simulink library "libturbines"  (R2025b)
settings: Solver=ode45  StartTime=0.0  StopTime=10.0  RelTol=1e-3  EnableMultiTasking=on
undefined symbols (not defined in the file): DiscIntNeverNeededParam, dt, faultOptions, noiseFlag
libraries: simulink x57, $bdroot x3
(part 3 of 5)

== system libturbines/Floating NREL5MW faulty/Controller ==
  P_dem [W] : Inport
  w_gen_meas [m/s] : Inport  Port=2
  beta_meas [deg] : Inport  Port=3
  Gain : Gain  Gain=[1 0 0]  Multiplication=Matrix(K*u) (u vector)
  Generator efficiency compensation : Gain  Gain=1/wt.ctrl.gen.effeciency
  Limit power to rated : Saturate  UpperLimit=wt.ctrl.p_rated  LowerLimit=0
  Measurement filter (low pass) : DiscreteStateSpace  A=wt.ctrl.alpha  B=1-wt.ctrl.alpha  C=wt.ctrl.alpha  D=1-wt.ctrl.alpha  InitialCondition=wt.ctrl.gen.ini  SampleTime=wt.ctrl.Ts
  Pitch controller : Subsystem  TreatAsAtomicUnit=on
  Rate Limiter : RateLimiter  RisingSlewLimit=wt.ctrl.torq.ratelim  FallingSlewLimit=-wt.ctrl.torq.ratelim  SampleTimeMode=inherited  InitialCondition=wt.ctrl.torq.ini
  Rated speed : Constant  Value=wt.ctrl.gen.rated
  Region check : Subsystem
  Sample output : ZeroOrderHold  SampleTime=wt.ctrl.Ts
  Sample power demand : ZeroOrderHold  SampleTime=wt.ctrl.Ts
  Saturation : Saturate  UpperLimit=wt.ctrl.torq.lim  LowerLimit=0
  Sum : Sum  Inputs=+-|
  Torque - speed lookup table : Lookup  InputValues=wt.ctrl.torq.wg  Table=wt.ctrl.torq.M  LookUpMeth=Interpolation-Use End Values  SaturateOnIntegerOverflow=off
  Zero-Order Hold : ZeroOrderHold  SampleTime=wt.ctrl.Ts
  beta_ref [deg] : Outport
  T_g_ref [W] : Outport  Port=2
  wires:
  Region check/2(Enable pitch controller) -> Pitch controller/Enable
  Sum/1 -> Pitch controller/1(w_gen_diff)
  Rated speed/1 -> Sum/1
  Sample power demand/1 -> Generator efficiency compensation/1
  Rate Limiter/1 -> Sample output/1
  Generator efficiency compensation/1 -> Limit power to rated/1
  Sample output/1 -> T_g_ref [W]/1
  Zero-Order Hold/1 -> beta_ref [deg]/1
  Limit power to rated/1 -> Region check/3(p_dem), Pitch controller/2(P_dem)
  Region check/1(Torque_ref) -> Saturation/1
  P_dem [W]/1 -> Sample power demand/1
  Torque - speed lookup table/1 -> Region check/1(Torque_dem)  "Desired Torque"
  Pitch controller/1(beta_ref [deg]) -> Gain/1, Zero-Order Hold/1
  Saturation/1 -> Rate Limiter/1
  Measurement filter (low pass)/1 -> Sum/2, Region check/2(w_gen), Torque - speed lookup table/1  "Filtered generator speed"
  w_gen_meas [m/s]/1 -> Measurement filter (low pass)/1
  Gain/1 -> Region check/4(pitch command)
  beta_meas [deg]/1 -> Pitch controller/3(beta_meas [deg])

== system libturbines/Floating NREL5MW faulty/Drive Train ==
  M_rot [Nm] : Inport
  M_gen [Nm] : Inport  Port=2
  Demux : Demux  Outputs=3
  Drive train dynamics : StateSpace  A=wt.dt.ssA  B=wt.dt.ssB  C=wt.dt.ssC  D=wt.dt.ssD  InitialCondition=[wt.rotor.ini;wt.gen.ini;0]
  Mux : Mux  Inputs=2
  w_rot [rad/s] : Outport
  w_gen [rad/s] : Outport  Port=2
  M_shaft [Nm] : Outport  Port=3
  wires:
  Mux/1 -> Drive train dynamics/1
  M_rot [Nm]/1 -> Mux/1
  M_gen [Nm]/1 -> Mux/2
  Drive train dynamics/1 -> Demux/1
  Demux/1 -> w_rot [rad/s]/1
  Demux/2 -> w_gen [rad/s]/1
  Demux/3 -> M_shaft [Nm]/1

== system libturbines/Floating NREL5MW faulty/Generator simple ==
  w_gen [rad/s] : Inport
  T_g_ref [W] : Inport  Port=2
  GenActFault : Inport  Port=3
  Constant : Constant  Value=wt.gen.timeconstant
  Delay : Delay  DelayLength=1  InitialCondition=0
  Delay1 : Delay  DelayLength=1  InitialCondition=0
  Demux : Demux  Outputs=2
  Divide1 : Product  Inputs=*/
  Generator efficiency : Gain  Gain=wt.gen.effeciency
  Generator fault : MATLAB Function  TreatAsAtomicUnit=on
  Generator fault type 3 : MATLAB Function  TreatAsAtomicUnit=on
  Multiply : Product  Inputs=**
  Product : Product
  Sum : Sum  Inputs=|+-
  Torque Integrator : Integrator  InitialCondition=wt.gen.torq.ini
  M_gen [Nm] : Outport
  P_out [W] : Outport  Port=2
  wires:
  Divide1/1 -> Torque Integrator/1
  Generator efficiency/1 -> P_out [W]/1
  Multiply/1 -> Generator efficiency/1
  T_g_ref [W]/1 -> Sum/1
  Torque Integrator/1 -> Generator fault/2(torque), Sum/2
  w_gen [rad/s]/1 -> Multiply/2
  GenActFault/1 -> Generator fault type 3/1(GenActFault)
  Generator fault type 3/1(out) -> Demux/1
  Demux/1 -> Generator fault/1(GenActFault)
  Generator fault/1(torque_real) -> Multiply/1, Delay/1, M_gen [Nm]/1
  Constant/1 -> Product/2
  Demux/2 -> Product/1
  Product/1 -> Divide1/2
  Sum/1 -> Divide1/1
  Delay/1 -> Generator fault/3(torque_prev)
  Generator fault/2(drift_aux_out) -> Delay1/1
  Delay1/1 -> Generator fault/4(drift_aux_in)

== system libturbines/Floating NREL5MW faulty/Hydrodynamics ==
  F_t [N] : Inport
  F_ex : Inport  Port=2
  Gain : Gain  Gain=plat.nF2pT  Multiplication=Matrix(K*u)
  Gain2 : Gain  Gain=plat.pM2nM_surge  Multiplication=Matrix(K*u)
  Gain3 : Gain  Gain=plat.pM2nM_pitch  Multiplication=Matrix(K*u)
  Platform hydrodynamics SS system : StateSpace  A=plat.HydSys.a  B=plat.HydSys.b  C=plat.HydSys.c  D=plat.HydSys.d  InitialCondition=0
  Sum : Sum  Inputs=++|
  Sum2 : Sum  Inputs=+|+
  v_nac_hyd [m/s] : Outport
  wires:
  F_ex/1 -> Sum/2
  Sum/1 -> Platform hydrodynamics SS system/1
  Sum2/1 -> v_nac_hyd [m/s]/1
  Platform hydrodynamics SS system/1 -> Gain3/1, Gain2/1
  Gain2/1 -> Sum2/1
  Gain3/1 -> Sum2/2
  Gain/1 -> Sum/1
  F_t [N]/1 -> Gain/1

== system libturbines/Floating NREL5MW faulty/Pitch Actuator ==
  beta_ref [deg] : Inport
  PitchActFault : Inport  Port=2
  Delay1 : Delay  DelayLength=1  InitialCondition=0
  Delay2 : Delay  DelayLength=1  InitialCondition=0
  Pitch actuator fault : MATLAB Function  TreatAsAtomicUnit=on
  Pitch subsystems : Subsystem
  beta [deg] : Outport
  wires:
  PitchActFault/1 -> Pitch subsystems/2(Fault type 5), Pitch actuator fault/3(PitchActFault)
  beta_ref [deg]/1 -> Pitch subsystems/1(beta_ref [deg])
  Pitch actuator fault/1(beta_real) -> Delay1/1, beta [deg]/1
  Pitch subsystems/1(beta [deg]) -> Pitch actuator fault/1(beta)
  Pitch actuator fault/2(drift_aux_out) -> Delay2/1
  Delay2/1 -> Pitch actuator fault/4(drift_aux_in)
  Delay1/1 -> Pitch actuator fault/2(beta_prev)

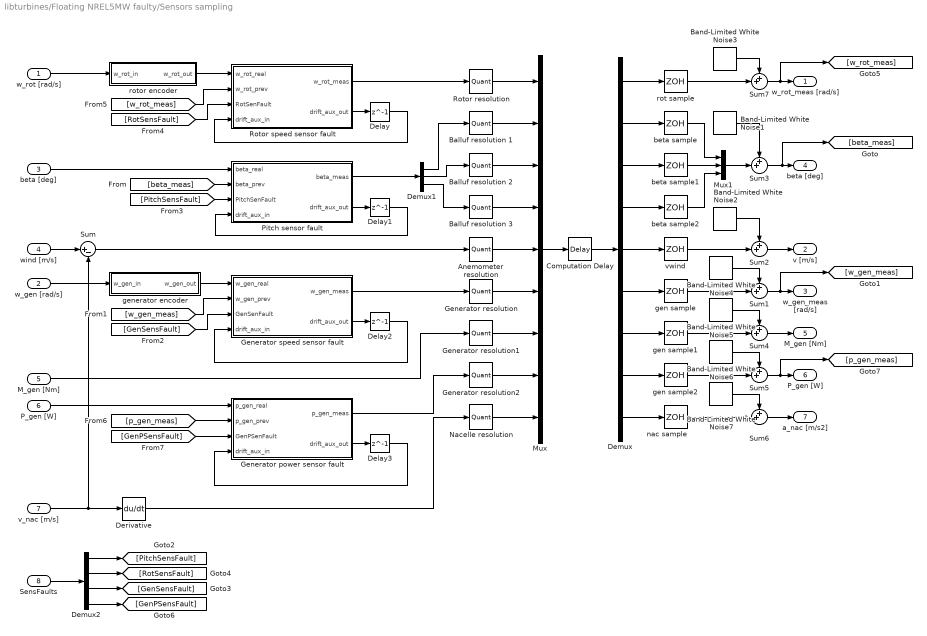
== system libturbines/Floating NREL5MW faulty/Sensors sampling ==
  "w_rot [rad/s] " : Inport
  w_gen [rad/s] : Inport  Port=2
  "beta [deg] " : Inport  Port=3
  wind [m/s] : Inport  Port=4
  "M_gen [Nm] " : Inport  Port=5
  "P_gen [W] " : Inport  Port=6
  "v_nac [m/s] " : Inport  Port=7
  SensFaults : Inport  Port=8
  Anemometer resolution : Quantizer  QuantizationInterval=wt.meas.aneres
  Balluf resolution 1 : Quantizer  QuantizationInterval=wt.meas.pitchres
  Balluf resolution 2 : Quantizer  QuantizationInterval=wt.meas.pitchres
  Balluf resolution 3 : Quantizer  QuantizationInterval=wt.meas.pitchres
  Band-Limited White Noise1 : simulink/Sources/Band-Limited White Noise  Cov=noiseFlag*wt.meas.pitchnoise  Ts=dt  seed=floor(10000*rand(1,3))
  Band-Limited White Noise2 : simulink/Sources/Band-Limited White Noise  Cov=noiseFlag*wt.meas.anenoise  Ts=dt  seed=floor(10000*rand(1))
  Band-Limited White Noise3 : simulink/Sources/Band-Limited White Noise  Cov=noiseFlag*wt.meas.rotSpdnoise  Ts=dt  seed=floor(10000*rand(1))
  Band-Limited White Noise4 : simulink/Sources/Band-Limited White Noise  Cov=noiseFlag*wt.meas.genSpdnoise  Ts=dt  seed=floor(10000*rand(1))
  Band-Limited White Noise5 : simulink/Sources/Band-Limited White Noise  Cov=noiseFlag*wt.meas.genTrqnoise  Ts=dt  seed=floor(10000*rand(1))
  Band-Limited White Noise6 : simulink/Sources/Band-Limited White Noise  Cov=noiseFlag*wt.meas.genPwrnoise  Ts=dt  seed=floor(10000*rand(1))
  Band-Limited White Noise7 : simulink/Sources/Band-Limited White Noise  Cov=noiseFlag*wt.meas.nacAccnoise  Ts=dt  seed=floor(10000*rand(1))
  Computation Delay : TransportDelay  DelayTime=wt.meas.delay  InitialOutput=[wt.rotor.ini wt.pitch.ini wt.pitch.ini wt.pitch.ini 0 wt.gen.ini 0 0 0]
  Delay{,1..3} (4 alike) : Delay  DelayLength=1  InitialCondition=0
  Demux : Demux  Outputs=9
  Demux1 : Demux  Outputs=3
  Demux2 : Demux
  Derivative : Derivative
  Generator power sensor fault : MATLAB Function  TreatAsAtomicUnit=on
  Generator resolution : Quantizer  QuantizationInterval=wt.meas.genres
  Generator resolution1 : Quantizer  QuantizationInterval=wt.meas.genres
  Generator resolution2 : Quantizer  QuantizationInterval=wt.meas.genres
  Generator speed sensor fault : MATLAB Function  TreatAsAtomicUnit=on
  Mux : Mux  Inputs=9
  Mux1 : Mux  Inputs=3
  Nacelle resolution : Quantizer  QuantizationInterval=wt.meas.nacres
  Pitch sensor fault : MATLAB Function  TreatAsAtomicUnit=on
  Rotor resolution : Quantizer  QuantizationInterval=wt.meas.rotres
  Rotor speed sensor fault : MATLAB Function  TreatAsAtomicUnit=on
  Sum : Sum  Inputs=|+-
  Sum{1..7} (7 alike) : Sum  Inputs=++|
  beta sample : ZeroOrderHold  SampleTime=wt.meas.Ts
  beta sample1 : ZeroOrderHold  SampleTime=wt.meas.Ts
  beta sample2 : ZeroOrderHold  SampleTime=wt.meas.Ts
  gen sample : ZeroOrderHold  SampleTime=wt.meas.Ts
  gen sample1 : ZeroOrderHold  SampleTime=wt.meas.Ts
  gen sample2 : ZeroOrderHold  SampleTime=wt.meas.Ts
  generator encoder : Subsystem
  nac sample : ZeroOrderHold  SampleTime=wt.meas.Ts
  rot sample : ZeroOrderHold  SampleTime=wt.meas.Ts
  rotor encoder : Subsystem
  vwind : ZeroOrderHold  SampleTime=wt.meas.Ts
  w_rot_meas [rad/s] : Outport  InitialOutput=0
  v [m/s] : Outport  Port=2  InitialOutput=0
  w_gen_meas [rad/s] : Outport  Port=3  InitialOutput=0
  beta [deg] : Outport  Port=4  InitialOutput=0
  M_gen [Nm] : Outport  Port=5  InitialOutput=0
  P_gen [W] : Outport  Port=6  InitialOutput=0
  a_nac [m/s2] : Outport  Port=7  InitialOutput=0
  wires:
  beta sample1/1 -> Mux1/2
  Demux1/1 -> Balluf resolution 1/1
  Rotor resolution/1 -> Mux/1
  Generator resolution/1 -> Mux/6
  Demux1/2 -> Balluf resolution 2/1
  Demux/6 -> gen sample/1
  Anemometer resolution/1 -> Mux/5
  Demux/5 -> vwind/1
  Mux/1 -> Computation Delay/1
  Computation Delay/1 -> Demux/1
  Demux1/3 -> Balluf resolution 3/1
  beta sample/1 -> Mux1/1
  Demux/1 -> rot sample/1
  beta sample2/1 -> Mux1/3
  Demux/2 -> beta sample/1
  Balluf resolution 1/1 -> Mux/2
  Pitch sensor fault/1(beta_meas) -> Demux1/1
  "beta [deg] "/1 -> Pitch sensor fault/1(beta_real)
  Demux/4 -> beta sample2/1
  Demux/3 -> beta sample1/1
  Balluf resolution 2/1 -> Mux/3
  Balluf resolution 3/1 -> Mux/4
  Generator speed sensor fault/1(w_gen_meas) -> Generator resolution/1
  [w_gen_meas] -> Generator speed sensor fault/2(w_gen_prev)
  [beta_meas] -> Pitch sensor fault/2(beta_prev)
  w_gen [rad/s]/1 -> generator encoder/1(w_gen_in)
  generator encoder/1(w_gen_out) -> Generator speed sensor fault/1(w_gen_real)
  "w_rot [rad/s] "/1 -> rotor encoder/1(w_rot_in)
  Rotor speed sensor fault/1(w_rot_meas) -> Rotor resolution/1
  rotor encoder/1(w_rot_out) -> Rotor speed sensor fault/1(w_rot_real)
  SensFaults/1 -> Demux2/1
  Demux2/1 -> [PitchSensFault]
  [GenSensFault] -> Generator speed sensor fault/3(GenSenFault)
  [PitchSensFault] -> Pitch sensor fault/3(PitchSenFault)
  [RotSensFault] -> Rotor speed sensor fault/3(RotSenFault)
  [w_rot_meas] -> Rotor speed sensor fault/2(w_rot_prev)
  Demux2/2 -> [RotSensFault]
  Demux2/3 -> [GenSensFault]
  Rotor speed sensor fault/2(drift_aux_out) -> Delay/1
  Delay/1 -> Rotor speed sensor fault/4(drift_aux_in)
  Pitch sensor fault/2(drift_aux_out) -> Delay1/1
  Delay1/1 -> Pitch sensor fault/4(drift_aux_in)
  Generator speed sensor fault/2(drift_aux_out) -> Delay2/1
  Delay2/1 -> Generator speed sensor fault/4(drift_aux_in)
  "M_gen [Nm] "/1 -> Generator resolution1/1
  "v_nac [m/s] "/1 -> Derivative/1, Sum/2
  Derivative/1 -> Nacelle resolution/1
  Generator resolution1/1 -> Mux/7
  Nacelle resolution/1 -> Mux/9
  Generator resolution2/1 -> Mux/8
  Band-Limited White Noise5/1 -> Sum4/1
  Sum4/1 -> M_gen [Nm]/1
  Sum6/1 -> a_nac [m/s2]/1
  Band-Limited White Noise7/1 -> Sum6/1
  Band-Limited White Noise6/1 -> Sum5/1
  nac sample/1 -> Sum6/2
  gen sample1/1 -> Sum4/2
  Sum5/1 -> [p_gen_meas], P_gen [W]/1
  gen sample2/1 -> Sum5/2
  Demux/7 -> gen sample1/1
  Demux/8 -> gen sample2/1
  Demux/9 -> nac sample/1
  Sum1/1 -> [w_gen_meas], w_gen_meas [rad/s]/1
  gen sample/1 -> Sum1/2
  Sum2/1 -> v [m/s]/1
  vwind/1 -> Sum2/2
  Mux1/1 -> Sum3/2
  Sum3/1 -> [beta_meas], beta [deg]/1
  rot sample/1 -> Sum7/2
  Sum7/1 -> [w_rot_meas], w_rot_meas [rad/s]/1
  Band-Limited White Noise4/1 -> Sum1/1
  Band-Limited White Noise2/1 -> Sum2/1
  Band-Limited White Noise1/1 -> Sum3/1
  Band-Limited White Noise3/1 -> Sum7/1
  Sum/1 -> Anemometer resolution/1
  wind [m/s]/1 -> Sum/1
  Demux2/4 -> [GenPSensFault]
  Delay3/1 -> Generator power sensor fault/4(drift_aux_in)
  [GenPSensFault] -> Generator power sensor fault/3(GenPSenFault)
  Generator power sensor fault/2(drift_aux_out) -> Delay3/1
  "P_gen [W] "/1 -> Generator power sensor fault/1(p_gen_real)
  Generator power sensor fault/1(p_gen_meas) -> Generator resolution2/1
  [p_gen_meas] -> Generator power sensor fault/2(p_gen_prev)

== system libturbines/Floating NREL5MW faulty/Tower deflection  ==
  F_t [N] : Inport
  F_t*h : Gain  Gain=wt.tower.height  SaturateOnIntegerOverflow=on  OutDataTypeStr=Inherit: Same as input  ParamDataTypeStr=Inherit: Same as input
  Tower1 : Subsystem  mask(Tower (thrustwise)){mtop=wt.top.mass, mtow=wt.tower.mass, ftowY=wt.tower.eigfreq, dampY=wt.tower.damp}
      mask prompts: mtop "Mass of towertop [kg]"; mtow "Aequivalent tower mass [kg]"; ftowY "Tower eigenfrequency [Hz]"; dampY "Damping coefficient"
      mask help: Thrustwise dynamics of the tower
      mask init: same as libturbines/Floating IEA15MW/Tower /Tower1
      mask Help: The thrustwise tower dynamics are modelled as a linear oscillator
  v_nac [m/s] : Outport
  M_tow [Nm] : Outport  Port=2
  wires:
  Tower1/2(F_tow [N]) -> F_t*h/1
  F_t*h/1 -> M_tow [Nm]/1
  F_t [N]/1 -> Tower1/1(FT [Nm])
  Tower1/1(vnac [m/s]) -> v_nac [m/s]/1

== system libturbines/Floating IEA15MW/Controller/Pitch controller ==
  w_gen_diff : Inport
  P_dem : Inport  Port=2
  beta_meas [deg] : Inport  Port=3
  Enable : EnablePort  StatesWhenEnabling=reset  PropagateVarSize=During execution
  Blade 1 controller : Subsystem
  beta_ref [deg] : Outport  OutputWhenDisabled=reset  InitialOutput=wt.ctrl.torq.beta
  wires:
  Blade 1 controller/1(beta_ref [deg]) -> beta_ref [deg]/1
  beta_meas [deg]/1 -> Blade 1 controller/3(beta_meas [deg])
  P_dem/1 -> Blade 1 controller/2(P_dem)
  w_gen_diff/1 -> Blade 1 controller/1(w_gen_diff)

== system libturbines/Floating IEA15MW/Controller/Region check ==
  Torque_dem : Inport
  w_gen : Inport  Port=2
  p_dem : Inport  Port=3
  pitch command : Inport  Port=4
  Demand limitation : RelationalOperator  Operator=<=  OutDataTypeStr=boolean  InputSameDT=off
  Divide : Product  Inputs=*/
  Enable Pitch control? : Logic  Operator=OR  Inputs=3  AllPortsSameDT=off  OutDataTypeStr=boolean
  Integer Delay : Delay  DelayLength=1
  Pitch actuator active last time? : simulink/Logic and Bit Operations/Compare To Constant  relop=>  const=wt.ctrl.torq.beta  OutDataTypeStr=uint8  ZeroCross=off
  Product : Product  RndMeth=Zero
  Region 3 speed? : simulink/Logic and Bit Operations/Compare To Constant  relop=>=  const=wt.ctrl.torq.r3  OutDataTypeStr=uint8  ZeroCross=off
  Switch Torque_ref : Switch  Threshold=1  SaturateOnIntegerOverflow=off  InputSameDT=off
  Torque_ref : Outport
  Enable pitch controller : Outport  Port=2
  wires:
  Divide/1 -> Switch Torque_ref/1
  Switch Torque_ref/1 -> Torque_ref/1
  Demand limitation/1 -> Enable Pitch control?/1
  p_dem/1 -> Divide/1, Demand limitation/1
  Torque_dem/1 -> Switch Torque_ref/3, Product/1
  Product/1 -> Demand limitation/2
  Enable Pitch control?/1 -> Switch Torque_ref/2, Enable pitch controller/1
  Integer Delay/1 -> Pitch actuator active last time?/1
  Region 3 speed?/1 -> Enable Pitch control?/2
  Pitch actuator active last time?/1 -> Enable Pitch control?/3
  w_gen/1 -> Product/2, Region 3 speed?/1, Divide/2
  pitch command/1 -> Integer Delay/1

== system libturbines/Floating IEA15MW/Sensors sampling/generator encoder ==
  w_gen_in : Inport
  Sum : Sum  Inputs=-+|
  gen Integrator : Integrator  InitialCondition=wt.gen.ini
  gen sensor time constant : Gain  Gain=1/wt.meas.gentau
  w_gen_out : Outport
  wires:
  gen Integrator/1 -> w_gen_out/1, Sum/1
  Sum/1 -> gen sensor time constant/1
  gen sensor time constant/1 -> gen Integrator/1
  w_gen_in/1 -> Sum/2

== system libturbines/Floating IEA15MW/Sensors sampling/rotor encoder ==
  w_rot_in : Inport
  Sum1 : Sum  Inputs=|+-
  gen Integrator1 : Integrator  InitialCondition=wt.rotor.ini
  gen sensor time constant1 : Gain  Gain=1/wt.meas.rottau
  w_rot_out : Outport
  wires:
  w_rot_in/1 -> Sum1/1
  gen Integrator1/1 -> w_rot_out/1, Sum1/2
  Sum1/1 -> gen sensor time constant1/1
  gen sensor time constant1/1 -> gen Integrator1/1

== system libturbines/Floating IEA15MW/Tower /Tower1 ==
  FT [Nm] : Inport
  Demux1 : Demux  Outputs=2
  Tower : StateSpace  A=A  B=B  C=C  D=D  InitialCondition=zeros(2,1)
  vnac [m/s] : Outport  InitialOutput=0
  F_tow [N] : Outport  Port=2  InitialOutput=0
  wires:
  Demux1/2 -> F_tow [N]/1
  FT [Nm]/1 -> Tower/1
  Demux1/1 -> vnac [m/s]/1
  Tower/1 -> Demux1/1

== system libturbines/Floating IEA15MW faulty/Aerodynamics/Blade 1 ==
  note: tip speed
      | [m/s]
  v_rot [m/s] : Inport
  beta [deg] : Inport  Port=2
  w_rot [rad/s] : Inport  Port=3
  C_P & C_T tables : Subsystem
  Gain : Gain  Gain=1/3
  Gain1 : Gain  Gain=1/3
  Gain2 : Gain  Gain=1/3
  Math Function : Math  Operator=square  SignedPower=on
  Product : Product  InputSameDT=on  SaturateOnIntegerOverflow=on  OutDataTypeStr=Inherit: Same as first input
  Product1 : Product  Inputs=**/  InputSameDT=on  SaturateOnIntegerOverflow=on  OutDataTypeStr=Inherit: Same as first input
  Product2 : Product  InputSameDT=on  SaturateOnIntegerOverflow=on  OutDataTypeStr=Inherit: Same as first input
  Product3 : Product  Inputs=/*  InputSameDT=on  SaturateOnIntegerOverflow=on  OutDataTypeStr=Inherit: Same as first input
  rho/2*A : Gain  Gain=env.rho*.5* pi * wt.rotor.radius^2  SaturateOnIntegerOverflow=on  OutDataTypeStr=Inherit: Same as input  ParamDataTypeStr=Inherit: Same as input
  rotor radius : Gain  Gain=wt.rotor.radius  SaturateOnIntegerOverflow=on  OutDataTypeStr=Inherit: Same as input  ParamDataTypeStr=Inherit: Same as input
  F_t [N] : Outport
  C_T : Outport  Port=2
  M_rot [Nm] : Outport  Port=3
  wires:
  Gain1/1 -> C_T/1
  Gain2/1 -> M_rot [Nm]/1
  Gain/1 -> F_t [N]/1
  Product/1 -> Gain/1
  Product1/1 -> Gain2/1
  beta [deg]/1 -> C_P & C_T tables/1(beta)
  Math Function/1 -> rho/2*A/1
  rotor radius/1 -> Product3/2
  v_rot [m/s]/1 -> Math Function/1, Product3/1, Product2/1
  w_rot [rad/s]/1 -> rotor radius/1, Product1/3
  Product2/1 -> Product1/2
  rho/2*A/1 -> Product2/2, Product/1
  Product3/1 -> C_P & C_T tables/2(lambda)
  C_P & C_T tables/1(C_T) -> Product/2, Gain1/1
  C_P & C_T tables/2(C_P) -> Product1/1

== system libturbines/Floating IEA15MW faulty/Aerodynamics/Blade 2 ==
  note: tip speed
      | [m/s]
  v_rot [m/s] : Inport
  beta [deg] : Inport  Port=2
  w_rot [rad/s] : Inport  Port=3
  C_P & C_T tables : Subsystem
  Gain : Gain  Gain=1/3
  Gain1 : Gain  Gain=1/3
  Gain2 : Gain  Gain=1/3
  Math Function : Math  Operator=square  SignedPower=on
  Product : Product  InputSameDT=on  SaturateOnIntegerOverflow=on  OutDataTypeStr=Inherit: Same as first input
  Product1 : Product  Inputs=**/  InputSameDT=on  SaturateOnIntegerOverflow=on  OutDataTypeStr=Inherit: Same as first input
  Product2 : Product  InputSameDT=on  SaturateOnIntegerOverflow=on  OutDataTypeStr=Inherit: Same as first input
  Product3 : Product  Inputs=/*  InputSameDT=on  SaturateOnIntegerOverflow=on  OutDataTypeStr=Inherit: Same as first input
  rho/2*A : Gain  Gain=env.rho*.5* pi * wt.rotor.radius^2  SaturateOnIntegerOverflow=on  OutDataTypeStr=Inherit: Same as input  ParamDataTypeStr=Inherit: Same as input
  rotor radius : Gain  Gain=wt.rotor.radius  SaturateOnIntegerOverflow=on  OutDataTypeStr=Inherit: Same as input  ParamDataTypeStr=Inherit: Same as input
  F_t [N] : Outport
  C_T : Outport  Port=2
  M_rot [Nm] : Outport  Port=3
  wires:
  Gain1/1 -> C_T/1
  Gain2/1 -> M_rot [Nm]/1
  Gain/1 -> F_t [N]/1
  Product/1 -> Gain/1
  Product1/1 -> Gain2/1
  beta [deg]/1 -> C_P & C_T tables/1(beta)
  Math Function/1 -> rho/2*A/1
  rotor radius/1 -> Product3/2
  v_rot [m/s]/1 -> Math Function/1, Product3/1, Product2/1
  w_rot [rad/s]/1 -> rotor radius/1, Product1/3
  Product2/1 -> Product1/2
  rho/2*A/1 -> Product2/2, Product/1
  Product3/1 -> C_P & C_T tables/2(lambda)
  C_P & C_T tables/1(C_T) -> Product/2, Gain1/1
  C_P & C_T tables/2(C_P) -> Product1/1

== system libturbines/Floating IEA15MW faulty/Aerodynamics/Blade 3 ==
  note: tip speed
      | [m/s]
  v_rot [m/s] : Inport
  beta [deg] : Inport  Port=2
  w_rot [rad/s] : Inport  Port=3
  C_P & C_T tables : Subsystem
  Gain : Gain  Gain=1/3
  Gain1 : Gain  Gain=1/3
  Gain2 : Gain  Gain=1/3
  Math Function : Math  Operator=square  SignedPower=on
  Product : Product  InputSameDT=on  SaturateOnIntegerOverflow=on  OutDataTypeStr=Inherit: Same as first input
  Product1 : Product  Inputs=**/  InputSameDT=on  SaturateOnIntegerOverflow=on  OutDataTypeStr=Inherit: Same as first input
  Product2 : Product  InputSameDT=on  SaturateOnIntegerOverflow=on  OutDataTypeStr=Inherit: Same as first input
  Product3 : Product  Inputs=/*  InputSameDT=on  SaturateOnIntegerOverflow=on  OutDataTypeStr=Inherit: Same as first input
  rho/2*A : Gain  Gain=env.rho*.5* pi * wt.rotor.radius^2  SaturateOnIntegerOverflow=on  OutDataTypeStr=Inherit: Same as input  ParamDataTypeStr=Inherit: Same as input
  rotor radius : Gain  Gain=wt.rotor.radius  SaturateOnIntegerOverflow=on  OutDataTypeStr=Inherit: Same as input  ParamDataTypeStr=Inherit: Same as input
  F_t [N] : Outport
  C_T : Outport  Port=2
  M_rot [Nm] : Outport  Port=3
  wires:
  Gain1/1 -> C_T/1
  Gain2/1 -> M_rot [Nm]/1
  Gain/1 -> F_t [N]/1
  Product/1 -> Gain/1
  Product1/1 -> Gain2/1
  beta [deg]/1 -> C_P & C_T tables/1(beta)
  Math Function/1 -> rho/2*A/1
  rotor radius/1 -> Product3/2
  v_rot [m/s]/1 -> Math Function/1, Product3/1, Product2/1
  w_rot [rad/s]/1 -> rotor radius/1, Product1/3
  Product2/1 -> Product1/2
  rho/2*A/1 -> Product2/2, Product/1
  Product3/1 -> C_P & C_T tables/2(lambda)
  C_P & C_T tables/1(C_T) -> Product/2, Gain1/1
  C_P & C_T tables/2(C_P) -> Product1/1

== system libturbines/Floating IEA15MW faulty/Controller/Pitch controller ==
  w_gen_diff : Inport
  P_dem : Inport  Port=2
  beta_meas [deg] : Inport  Port=3
  Enable : EnablePort  StatesWhenEnabling=reset  PropagateVarSize=During execution
  Blade 1 controller : Subsystem
  Blade 2 controller : Subsystem
  Blade 3 controller : Subsystem
  Demux : Demux  Outputs=3
  Mux : Mux  Inputs=3
  beta_ref [deg] : Outport  OutputWhenDisabled=reset  InitialOutput=wt.ctrl.torq.beta
  wires:
  Mux/1 -> beta_ref [deg]/1
  w_gen_diff/1 -> Blade 1 controller/1(w_gen_diff), Blade 2 controller/1(w_gen_diff), Blade 3 controller/1(w_gen_diff)
  P_dem/1 -> Blade 1 controller/2(P_dem), Blade 2 controller/2(P_dem), Blade 3 controller/2(P_dem)
  Demux/1 -> Blade 1 controller/3(beta_meas [deg])
  Blade 1 controller/1(beta_ref [deg]) -> Mux/1
  Demux/2 -> Blade 2 controller/3(beta_meas [deg])
  beta_meas [deg]/1 -> Demux/1
  Blade 3 controller/1(beta_ref [deg]) -> Mux/3
  Demux/3 -> Blade 3 controller/3(beta_meas [deg])
  Blade 2 controller/1(beta_ref [deg]) -> Mux/2

== system libturbines/Floating IEA15MW faulty/Controller/Region check ==
  Torque_dem : Inport
  w_gen : Inport  Port=2
  p_dem : Inport  Port=3
  pitch command : Inport  Port=4
  Demand limitation : RelationalOperator  Operator=<=  OutDataTypeStr=boolean  InputSameDT=off
  Divide : Product  Inputs=*/
  Enable Pitch control? : Logic  Operator=OR  Inputs=3  AllPortsSameDT=off  OutDataTypeStr=boolean
  Integer Delay : Delay  DelayLength=1
  Pitch actuator active last time? : simulink/Logic and Bit Operations/Compare To Constant  relop=>  const=wt.ctrl.torq.beta  OutDataTypeStr=uint8  ZeroCross=off
  Product : Product  RndMeth=Zero
  Region 3 speed? : simulink/Logic and Bit Operations/Compare To Constant  relop=>=  const=wt.ctrl.torq.r3  OutDataTypeStr=uint8  ZeroCross=off
  Switch Torque_ref : Switch  Threshold=1  SaturateOnIntegerOverflow=off  InputSameDT=off
  Torque_ref : Outport
  Enable pitch controller : Outport  Port=2
  wires:
  pitch command/1 -> Integer Delay/1
  w_gen/1 -> Divide/2, Region 3 speed?/1, Product/2
  Pitch actuator active last time?/1 -> Enable Pitch control?/3
  Region 3 speed?/1 -> Enable Pitch control?/2
  Integer Delay/1 -> Pitch actuator active last time?/1
  Enable Pitch control?/1 -> Enable pitch controller/1, Switch Torque_ref/2
  Product/1 -> Demand limitation/2
  Torque_dem/1 -> Product/1, Switch Torque_ref/3
  p_dem/1 -> Demand limitation/1, Divide/1
  Demand limitation/1 -> Enable Pitch control?/1
  Switch Torque_ref/1 -> Torque_ref/1
  Divide/1 -> Switch Torque_ref/1

== system libturbines/Floating IEA15MW faulty/Pitch Actuator/Pitch subsystems ==
  beta_ref [deg] : Inport
  Fault type 5 : Inport  Port=2
  Demux2 : Demux  Outputs=3
  Mux1 : Mux  Inputs=3
  Pitch system B1 : StateSpace  A=wt.pitch.ssA  B=wt.pitch.ssB  C=wt.pitch.ssC  D=wt.pitch.ssD  InitialCondition=0
  Pitch system B2 : StateSpace  A=wt.pitch.ssA  B=wt.pitch.ssB  C=wt.pitch.ssC  D=wt.pitch.ssD  InitialCondition=0
  Pitch system B3 : Subsystem
  beta [deg] : Outport
  wires:
  Demux2/2 -> Pitch system B2/1
  Demux2/1 -> Pitch system B1/1
  Pitch system B1/1 -> Mux1/1
  Pitch system B2/1 -> Mux1/2
  Mux1/1 -> beta [deg]/1
  beta_ref [deg]/1 -> Demux2/1
  Fault type 5/1 -> Pitch system B3/2(fault 5)
  Demux2/3 -> Pitch system B3/1(beta_ref [deg])
  Pitch system B3/1(beta [deg]) -> Mux1/3

== system libturbines/Floating IEA15MW faulty/Sensors sampling/generator encoder ==
  w_gen_in : Inport
  Sum : Sum  Inputs=-+|
  gen Integrator : Integrator  InitialCondition=wt.gen.ini
  gen sensor time constant : Gain  Gain=1/wt.meas.gentau
  w_gen_out : Outport
  wires:
  w_gen_in/1 -> Sum/2
  gen sensor time constant/1 -> gen Integrator/1
  Sum/1 -> gen sensor time constant/1
  gen Integrator/1 -> Sum/1, w_gen_out/1

== system libturbines/Floating IEA15MW faulty/Sensors sampling/rotor encoder ==
  w_rot_in : Inport
  Sum1 : Sum  Inputs=|+-
  gen Integrator1 : Integrator  InitialCondition=wt.rotor.ini
  gen sensor time constant1 : Gain  Gain=1/wt.meas.rottau
  w_rot_out : Outport
  wires:
  gen sensor time constant1/1 -> gen Integrator1/1
  Sum1/1 -> gen sensor time constant1/1
  gen Integrator1/1 -> Sum1/2, w_rot_out/1
  w_rot_in/1 -> Sum1/1

== system libturbines/Floating IEA15MW faulty/Tower deflection /Tower1 ==
  FT [Nm] : Inport
  Demux1 : Demux  Outputs=2
  Tower : StateSpace  A=A  B=B  C=C  D=D  InitialCondition=zeros(2,1)
  vnac [m/s] : Outport  InitialOutput=0
  F_tow [N] : Outport  Port=2  InitialOutput=0
  wires:
  Tower/1 -> Demux1/1
  Demux1/1 -> vnac [m/s]/1
  FT [Nm]/1 -> Tower/1
  Demux1/2 -> F_tow [N]/1

== system libturbines/Floating IEA3.4MW/Controller/Pitch controller ==
  w_gen_diff : Inport
  P_dem : Inport  Port=2
  beta_meas [deg] : Inport  Port=3
  Enable : EnablePort  StatesWhenEnabling=reset  PropagateVarSize=During execution
  Blade 1 controller : Subsystem
  beta_ref [deg] : Outport  OutputWhenDisabled=reset  InitialOutput=wt.ctrl.torq.beta
  wires:
  Blade 1 controller/1(beta_ref [deg]) -> beta_ref [deg]/1
  beta_meas [deg]/1 -> Blade 1 controller/3(beta_meas [deg])
  P_dem/1 -> Blade 1 controller/2(P_dem)
  w_gen_diff/1 -> Blade 1 controller/1(w_gen_diff)

== system libturbines/Floating IEA3.4MW/Controller/Region check ==
  Torque_dem : Inport
  w_gen : Inport  Port=2
  p_dem : Inport  Port=3
  pitch command : Inport  Port=4
  Demand limitation : RelationalOperator  Operator=<=  OutDataTypeStr=boolean  InputSameDT=off
  Divide : Product  Inputs=*/
  Enable Pitch control? : Logic  Operator=OR  Inputs=3  AllPortsSameDT=off  OutDataTypeStr=boolean
  Integer Delay : Delay  DelayLength=1
  Pitch actuator active last time? : simulink/Logic and Bit Operations/Compare To Constant  relop=>  const=wt.ctrl.torq.beta  OutDataTypeStr=uint8  ZeroCross=off
  Product : Product  RndMeth=Zero
  Region 3 speed? : simulink/Logic and Bit Operations/Compare To Constant  relop=>=  const=wt.ctrl.torq.r3  OutDataTypeStr=uint8  ZeroCross=off
  Switch Torque_ref : Switch  Threshold=1  SaturateOnIntegerOverflow=off  InputSameDT=off
  Torque_ref : Outport
  Enable pitch controller : Outport  Port=2
  wires:
  Divide/1 -> Switch Torque_ref/1
  Switch Torque_ref/1 -> Torque_ref/1
  Demand limitation/1 -> Enable Pitch control?/1
  p_dem/1 -> Divide/1, Demand limitation/1
  Torque_dem/1 -> Switch Torque_ref/3, Product/1
  Product/1 -> Demand limitation/2
  Enable Pitch control?/1 -> Switch Torque_ref/2, Enable pitch controller/1
  Integer Delay/1 -> Pitch actuator active last time?/1
  Region 3 speed?/1 -> Enable Pitch control?/2
  Pitch actuator active last time?/1 -> Enable Pitch control?/3
  w_gen/1 -> Product/2, Region 3 speed?/1, Divide/2
  pitch command/1 -> Integer Delay/1

== system libturbines/Floating IEA3.4MW/Sensors sampling/generator encoder ==
  w_gen_in : Inport
  Sum : Sum  Inputs=-+|
  gen Integrator : Integrator  InitialCondition=wt.gen.ini
  gen sensor time constant : Gain  Gain=1/wt.meas.gentau
  w_gen_out : Outport
  wires:
  gen Integrator/1 -> w_gen_out/1, Sum/1
  Sum/1 -> gen sensor time constant/1
  gen sensor time constant/1 -> gen Integrator/1
  w_gen_in/1 -> Sum/2

== system libturbines/Floating IEA3.4MW/Sensors sampling/rotor encoder ==
  w_rot_in : Inport
  Sum1 : Sum  Inputs=|+-
  gen Integrator1 : Integrator  InitialCondition=wt.rotor.ini
  gen sensor time constant1 : Gain  Gain=1/wt.meas.rottau
  w_rot_out : Outport
  wires:
  w_rot_in/1 -> Sum1/1
  gen Integrator1/1 -> w_rot_out/1, Sum1/2
  Sum1/1 -> gen sensor time constant1/1
  gen sensor time constant1/1 -> gen Integrator1/1

== system libturbines/Floating IEA3.4MW/Tower /Tower1 ==
  FT [Nm] : Inport
  Demux1 : Demux  Outputs=2
  Tower : StateSpace  A=A  B=B  C=C  D=D  InitialCondition=zeros(2,1)
  vnac [m/s] : Outport  InitialOutput=0
  F_tow [N] : Outport  Port=2  InitialOutput=0
  wires:
  Demux1/2 -> F_tow [N]/1
  FT [Nm]/1 -> Tower/1
  Demux1/1 -> vnac [m/s]/1
  Tower/1 -> Demux1/1

== system libturbines/Floating IEA3.4MW faulty/Aerodynamics/Blade 1 ==
  note: tip speed
      | [m/s]
  v_rot [m/s] : Inport
  beta [deg] : Inport  Port=2
  w_rot [rad/s] : Inport  Port=3
  C_P & C_T tables : Subsystem
  Gain : Gain  Gain=1/3
  Gain1 : Gain  Gain=1/3
  Gain2 : Gain  Gain=1/3
  Math Function : Math  Operator=square  SignedPower=on
  Product : Product  InputSameDT=on  SaturateOnIntegerOverflow=on  OutDataTypeStr=Inherit: Same as first input
  Product1 : Product  Inputs=**/  InputSameDT=on  SaturateOnIntegerOverflow=on  OutDataTypeStr=Inherit: Same as first input
  Product2 : Product  InputSameDT=on  SaturateOnIntegerOverflow=on  OutDataTypeStr=Inherit: Same as first input
  Product3 : Product  Inputs=/*  InputSameDT=on  SaturateOnIntegerOverflow=on  OutDataTypeStr=Inherit: Same as first input
  rho/2*A : Gain  Gain=env.rho*.5* pi * wt.rotor.radius^2  SaturateOnIntegerOverflow=on  OutDataTypeStr=Inherit: Same as input  ParamDataTypeStr=Inherit: Same as input
  rotor radius : Gain  Gain=wt.rotor.radius  SaturateOnIntegerOverflow=on  OutDataTypeStr=Inherit: Same as input  ParamDataTypeStr=Inherit: Same as input
  F_t [N] : Outport
  C_T : Outport  Port=2
  M_rot [Nm] : Outport  Port=3
  wires:
  Gain1/1 -> C_T/1
  Gain2/1 -> M_rot [Nm]/1
  Gain/1 -> F_t [N]/1
  Product/1 -> Gain/1
  Product1/1 -> Gain2/1
  beta [deg]/1 -> C_P & C_T tables/1(beta)
  Math Function/1 -> rho/2*A/1
  rotor radius/1 -> Product3/2
  v_rot [m/s]/1 -> Math Function/1, Product3/1, Product2/1
  w_rot [rad/s]/1 -> rotor radius/1, Product1/3
  Product2/1 -> Product1/2
  rho/2*A/1 -> Product2/2, Product/1
  Product3/1 -> C_P & C_T tables/2(lambda)
  C_P & C_T tables/1(C_T) -> Product/2, Gain1/1
  C_P & C_T tables/2(C_P) -> Product1/1

== system libturbines/Floating IEA3.4MW faulty/Aerodynamics/Blade 2 ==
  note: tip speed
      | [m/s]
  v_rot [m/s] : Inport
  beta [deg] : Inport  Port=2
  w_rot [rad/s] : Inport  Port=3
  C_P & C_T tables : Subsystem
  Gain : Gain  Gain=1/3
  Gain1 : Gain  Gain=1/3
  Gain2 : Gain  Gain=1/3
  Math Function : Math  Operator=square  SignedPower=on
  Product : Product  InputSameDT=on  SaturateOnIntegerOverflow=on  OutDataTypeStr=Inherit: Same as first input
  Product1 : Product  Inputs=**/  InputSameDT=on  SaturateOnIntegerOverflow=on  OutDataTypeStr=Inherit: Same as first input
  Product2 : Product  InputSameDT=on  SaturateOnIntegerOverflow=on  OutDataTypeStr=Inherit: Same as first input
  Product3 : Product  Inputs=/*  InputSameDT=on  SaturateOnIntegerOverflow=on  OutDataTypeStr=Inherit: Same as first input
  rho/2*A : Gain  Gain=env.rho*.5* pi * wt.rotor.radius^2  SaturateOnIntegerOverflow=on  OutDataTypeStr=Inherit: Same as input  ParamDataTypeStr=Inherit: Same as input
  rotor radius : Gain  Gain=wt.rotor.radius  SaturateOnIntegerOverflow=on  OutDataTypeStr=Inherit: Same as input  ParamDataTypeStr=Inherit: Same as input
  F_t [N] : Outport
  C_T : Outport  Port=2
  M_rot [Nm] : Outport  Port=3
  wires:
  Gain1/1 -> C_T/1
  Gain2/1 -> M_rot [Nm]/1
  Gain/1 -> F_t [N]/1
  Product/1 -> Gain/1
  Product1/1 -> Gain2/1
  beta [deg]/1 -> C_P & C_T tables/1(beta)
  Math Function/1 -> rho/2*A/1
  rotor radius/1 -> Product3/2
  v_rot [m/s]/1 -> Math Function/1, Product3/1, Product2/1
  w_rot [rad/s]/1 -> rotor radius/1, Product1/3
  Product2/1 -> Product1/2
  rho/2*A/1 -> Product2/2, Product/1
  Product3/1 -> C_P & C_T tables/2(lambda)
  C_P & C_T tables/1(C_T) -> Product/2, Gain1/1
  C_P & C_T tables/2(C_P) -> Product1/1

== system libturbines/Floating IEA3.4MW faulty/Aerodynamics/Blade 3 ==
  note: tip speed
      | [m/s]
  v_rot [m/s] : Inport
  beta [deg] : Inport  Port=2
  w_rot [rad/s] : Inport  Port=3
  C_P & C_T tables : Subsystem
  Gain : Gain  Gain=1/3
  Gain1 : Gain  Gain=1/3
  Gain2 : Gain  Gain=1/3
  Math Function : Math  Operator=square  SignedPower=on
  Product : Product  InputSameDT=on  SaturateOnIntegerOverflow=on  OutDataTypeStr=Inherit: Same as first input
  Product1 : Product  Inputs=**/  InputSameDT=on  SaturateOnIntegerOverflow=on  OutDataTypeStr=Inherit: Same as first input
  Product2 : Product  InputSameDT=on  SaturateOnIntegerOverflow=on  OutDataTypeStr=Inherit: Same as first input
  Product3 : Product  Inputs=/*  InputSameDT=on  SaturateOnIntegerOverflow=on  OutDataTypeStr=Inherit: Same as first input
  rho/2*A : Gain  Gain=env.rho*.5* pi * wt.rotor.radius^2  SaturateOnIntegerOverflow=on  OutDataTypeStr=Inherit: Same as input  ParamDataTypeStr=Inherit: Same as input
  rotor radius : Gain  Gain=wt.rotor.radius  SaturateOnIntegerOverflow=on  OutDataTypeStr=Inherit: Same as input  ParamDataTypeStr=Inherit: Same as input
  F_t [N] : Outport
  C_T : Outport  Port=2
  M_rot [Nm] : Outport  Port=3
  wires:
  Gain1/1 -> C_T/1
  Gain2/1 -> M_rot [Nm]/1
  Gain/1 -> F_t [N]/1
  Product/1 -> Gain/1
  Product1/1 -> Gain2/1
  beta [deg]/1 -> C_P & C_T tables/1(beta)
  Math Function/1 -> rho/2*A/1
  rotor radius/1 -> Product3/2
  v_rot [m/s]/1 -> Math Function/1, Product3/1, Product2/1
  w_rot [rad/s]/1 -> rotor radius/1, Product1/3
  Product2/1 -> Product1/2
  rho/2*A/1 -> Product2/2, Product/1
  Product3/1 -> C_P & C_T tables/2(lambda)
  C_P & C_T tables/1(C_T) -> Product/2, Gain1/1
  C_P & C_T tables/2(C_P) -> Product1/1

== system libturbines/Floating IEA3.4MW faulty/Controller/Pitch controller ==
  w_gen_diff : Inport
  P_dem : Inport  Port=2
  beta_meas [deg] : Inport  Port=3
  Enable : EnablePort  StatesWhenEnabling=reset  PropagateVarSize=During execution
  Blade 1 controller : Subsystem
  Blade 2 controller : Subsystem
  Blade 3 controller : Subsystem
  Demux : Demux  Outputs=3
  Mux : Mux  Inputs=3
  beta_ref [deg] : Outport  OutputWhenDisabled=reset  InitialOutput=wt.ctrl.torq.beta
  wires:
  Mux/1 -> beta_ref [deg]/1
  w_gen_diff/1 -> Blade 1 controller/1(w_gen_diff), Blade 2 controller/1(w_gen_diff), Blade 3 controller/1(w_gen_diff)
  P_dem/1 -> Blade 1 controller/2(P_dem), Blade 2 controller/2(P_dem), Blade 3 controller/2(P_dem)
  Demux/1 -> Blade 1 controller/3(beta_meas [deg])
  Blade 1 controller/1(beta_ref [deg]) -> Mux/1
  Demux/2 -> Blade 2 controller/3(beta_meas [deg])
  beta_meas [deg]/1 -> Demux/1
  Blade 3 controller/1(beta_ref [deg]) -> Mux/3
  Demux/3 -> Blade 3 controller/3(beta_meas [deg])
  Blade 2 controller/1(beta_ref [deg]) -> Mux/2

== system libturbines/Floating IEA3.4MW faulty/Controller/Region check ==
  Torque_dem : Inport
  w_gen : Inport  Port=2
  p_dem : Inport  Port=3
  pitch command : Inport  Port=4
  Demand limitation : RelationalOperator  Operator=<=  OutDataTypeStr=boolean  InputSameDT=off
  Divide : Product  Inputs=*/
  Enable Pitch control? : Logic  Operator=OR  Inputs=3  AllPortsSameDT=off  OutDataTypeStr=boolean
  Integer Delay : Delay  DelayLength=1
  Pitch actuator active last time? : simulink/Logic and Bit Operations/Compare To Constant  relop=>  const=wt.ctrl.torq.beta  OutDataTypeStr=uint8  ZeroCross=off
  Product : Product  RndMeth=Zero
  Region 3 speed? : simulink/Logic and Bit Operations/Compare To Constant  relop=>=  const=wt.ctrl.torq.r3  OutDataTypeStr=uint8  ZeroCross=off
  Switch Torque_ref : Switch  Threshold=1  SaturateOnIntegerOverflow=off  InputSameDT=off
  Torque_ref : Outport
  Enable pitch controller : Outport  Port=2
  wires:
  pitch command/1 -> Integer Delay/1
  w_gen/1 -> Divide/2, Region 3 speed?/1, Product/2
  Pitch actuator active last time?/1 -> Enable Pitch control?/3
  Region 3 speed?/1 -> Enable Pitch control?/2
  Integer Delay/1 -> Pitch actuator active last time?/1
  Enable Pitch control?/1 -> Enable pitch controller/1, Switch Torque_ref/2
  Product/1 -> Demand limitation/2
  Torque_dem/1 -> Product/1, Switch Torque_ref/3
  p_dem/1 -> Demand limitation/1, Divide/1
  Demand limitation/1 -> Enable Pitch control?/1
  Switch Torque_ref/1 -> Torque_ref/1
  Divide/1 -> Switch Torque_ref/1

== system libturbines/Floating IEA3.4MW faulty/Pitch Actuator/Pitch subsystems ==
  beta_ref [deg] : Inport
  Fault type 5 : Inport  Port=2
  Demux2 : Demux  Outputs=3
  Mux1 : Mux  Inputs=3
  Pitch system B1 : StateSpace  A=wt.pitch.ssA  B=wt.pitch.ssB  C=wt.pitch.ssC  D=wt.pitch.ssD  InitialCondition=0
  Pitch system B2 : StateSpace  A=wt.pitch.ssA  B=wt.pitch.ssB  C=wt.pitch.ssC  D=wt.pitch.ssD  InitialCondition=0
  Pitch system B3 : Subsystem
  beta [deg] : Outport
  wires:
  Demux2/2 -> Pitch system B2/1
  Demux2/1 -> Pitch system B1/1
  Pitch system B1/1 -> Mux1/1
  Pitch system B2/1 -> Mux1/2
  Mux1/1 -> beta [deg]/1
  beta_ref [deg]/1 -> Demux2/1
  Fault type 5/1 -> Pitch system B3/2(fault 5)
  Demux2/3 -> Pitch system B3/1(beta_ref [deg])
  Pitch system B3/1(beta [deg]) -> Mux1/3

== system libturbines/Floating IEA3.4MW faulty/Sensors sampling/generator encoder ==
  w_gen_in : Inport
  Sum : Sum  Inputs=-+|
  gen Integrator : Integrator  InitialCondition=wt.gen.ini
  gen sensor time constant : Gain  Gain=1/wt.meas.gentau
  w_gen_out : Outport
  wires:
  w_gen_in/1 -> Sum/2
  gen sensor time constant/1 -> gen Integrator/1
  Sum/1 -> gen sensor time constant/1
  gen Integrator/1 -> Sum/1, w_gen_out/1

== system libturbines/Floating IEA3.4MW faulty/Sensors sampling/rotor encoder ==
  w_rot_in : Inport
  Sum1 : Sum  Inputs=|+-
  gen Integrator1 : Integrator  InitialCondition=wt.rotor.ini
  gen sensor time constant1 : Gain  Gain=1/wt.meas.rottau
  w_rot_out : Outport
  wires:
  gen sensor time constant1/1 -> gen Integrator1/1
  Sum1/1 -> gen sensor time constant1/1
  gen Integrator1/1 -> Sum1/2, w_rot_out/1
  w_rot_in/1 -> Sum1/1

== system libturbines/Floating IEA3.4MW faulty/Tower deflection /Tower1 ==
  FT [Nm] : Inport
  Demux1 : Demux  Outputs=2
  Tower : StateSpace  A=A  B=B  C=C  D=D  InitialCondition=zeros(2,1)
  vnac [m/s] : Outport  InitialOutput=0
  F_tow [N] : Outport  Port=2  InitialOutput=0
  wires:
  Tower/1 -> Demux1/1
  Demux1/1 -> vnac [m/s]/1
  FT [Nm]/1 -> Tower/1
  Demux1/2 -> F_tow [N]/1

== system libturbines/Floating NREL5MW/Controller/Pitch controller ==
  w_gen_diff : Inport
  P_dem : Inport  Port=2
  beta_meas [deg] : Inport  Port=3
  Enable : EnablePort  StatesWhenEnabling=reset  PropagateVarSize=During execution
  Blade 1 controller : Subsystem
  beta_ref [deg] : Outport  OutputWhenDisabled=reset  InitialOutput=wt.ctrl.torq.beta
  wires:
  w_gen_diff/1 -> Blade 1 controller/1(w_gen_diff)
  P_dem/1 -> Blade 1 controller/2(P_dem)
  beta_meas [deg]/1 -> Blade 1 controller/3(beta_meas [deg])
  Blade 1 controller/1(beta_ref [deg]) -> beta_ref [deg]/1

== system libturbines/Floating NREL5MW/Controller/Region check ==
  Torque_dem : Inport
  w_gen : Inport  Port=2
  p_dem : Inport  Port=3
  pitch command : Inport  Port=4
  Demand limitation : RelationalOperator  Operator=<=  OutDataTypeStr=boolean  InputSameDT=off
  Divide : Product  Inputs=*/
  Enable Pitch control? : Logic  Operator=OR  Inputs=3  AllPortsSameDT=off  OutDataTypeStr=boolean
  Integer Delay : Delay  DelayLength=1
  Pitch actuator active last time? : simulink/Logic and Bit Operations/Compare To Constant  relop=>  const=wt.ctrl.torq.beta  OutDataTypeStr=uint8  ZeroCross=off
  Product : Product  RndMeth=Zero
  Region 3 speed? : simulink/Logic and Bit Operations/Compare To Constant  relop=>=  const=wt.ctrl.torq.r3  OutDataTypeStr=uint8  ZeroCross=off
  Switch Torque_ref : Switch  Threshold=1  SaturateOnIntegerOverflow=off  InputSameDT=off
  Torque_ref : Outport
  Enable pitch controller : Outport  Port=2
  wires:
  pitch command/1 -> Integer Delay/1
  w_gen/1 -> Divide/2, Region 3 speed?/1, Product/2
  Pitch actuator active last time?/1 -> Enable Pitch control?/3
  Region 3 speed?/1 -> Enable Pitch control?/2
  Integer Delay/1 -> Pitch actuator active last time?/1
  Enable Pitch control?/1 -> Enable pitch controller/1, Switch Torque_ref/2
  Product/1 -> Demand limitation/2
  Torque_dem/1 -> Product/1, Switch Torque_ref/3
  p_dem/1 -> Demand limitation/1, Divide/1
  Demand limitation/1 -> Enable Pitch control?/1
  Switch Torque_ref/1 -> Torque_ref/1
  Divide/1 -> Switch Torque_ref/1

== system libturbines/Floating NREL5MW/Sensors sampling/generator encoder ==
  w_gen_in : Inport
  Sum : Sum  Inputs=-+|
  gen Integrator : Integrator  InitialCondition=wt.gen.ini
  gen sensor time constant : Gain  Gain=1/wt.meas.gentau
  w_gen_out : Outport
  wires:
  w_gen_in/1 -> Sum/2
  gen sensor time constant/1 -> gen Integrator/1
  Sum/1 -> gen sensor time constant/1
  gen Integrator/1 -> Sum/1, w_gen_out/1

== system libturbines/Floating NREL5MW/Sensors sampling/rotor encoder ==
  w_rot_in : Inport
  Sum1 : Sum  Inputs=|+-
  gen Integrator1 : Integrator  InitialCondition=wt.rotor.ini
  gen sensor time constant1 : Gain  Gain=1/wt.meas.rottau
  w_rot_out : Outport
  wires:
  gen sensor time constant1/1 -> gen Integrator1/1
  Sum1/1 -> gen sensor time constant1/1
  gen Integrator1/1 -> Sum1/2, w_rot_out/1
  w_rot_in/1 -> Sum1/1

== system libturbines/Floating NREL5MW/Tower /Tower1 ==
  FT [Nm] : Inport
  Demux1 : Demux  Outputs=2
  Tower : StateSpace  A=A  B=B  C=C  D=D  InitialCondition=zeros(2,1)
  vnac [m/s] : Outport  InitialOutput=0
  F_tow [N] : Outport  Port=2  InitialOutput=0
  wires:
  Tower/1 -> Demux1/1
  Demux1/1 -> vnac [m/s]/1
  FT [Nm]/1 -> Tower/1
  Demux1/2 -> F_tow [N]/1

== system libturbines/Floating NREL5MW faulty/Aerodynamics/Blade 1 ==
  note: tip speed
      | [m/s]
  v_rot [m/s] : Inport
  beta [deg] : Inport  Port=2
  w_rot [rad/s] : Inport  Port=3
  C_P & C_T tables : Subsystem
  Gain : Gain  Gain=1/3
  Gain1 : Gain  Gain=1/3
  Gain2 : Gain  Gain=1/3
  Math Function : Math  Operator=square  SignedPower=on
  Product : Product  InputSameDT=on  SaturateOnIntegerOverflow=on  OutDataTypeStr=Inherit: Same as first input
  Product1 : Product  Inputs=**/  InputSameDT=on  SaturateOnIntegerOverflow=on  OutDataTypeStr=Inherit: Same as first input
  Product2 : Product  InputSameDT=on  SaturateOnIntegerOverflow=on  OutDataTypeStr=Inherit: Same as first input
  Product3 : Product  Inputs=/*  InputSameDT=on  SaturateOnIntegerOverflow=on  OutDataTypeStr=Inherit: Same as first input
  rho/2*A : Gain  Gain=env.rho*.5* pi * wt.rotor.radius^2  SaturateOnIntegerOverflow=on  OutDataTypeStr=Inherit: Same as input  ParamDataTypeStr=Inherit: Same as input
  rotor radius : Gain  Gain=wt.rotor.radius  SaturateOnIntegerOverflow=on  OutDataTypeStr=Inherit: Same as input  ParamDataTypeStr=Inherit: Same as input
  F_t [N] : Outport
  C_T : Outport  Port=2
  M_rot [Nm] : Outport  Port=3
  wires:
  C_P & C_T tables/2(C_P) -> Product1/1
  C_P & C_T tables/1(C_T) -> Gain1/1, Product/2
  Product3/1 -> C_P & C_T tables/2(lambda)
  rho/2*A/1 -> Product/1, Product2/2
  Product2/1 -> Product1/2
  w_rot [rad/s]/1 -> Product1/3, rotor radius/1
  v_rot [m/s]/1 -> Product2/1, Product3/1, Math Function/1
  rotor radius/1 -> Product3/2
  Math Function/1 -> rho/2*A/1
  beta [deg]/1 -> C_P & C_T tables/1(beta)
  Product1/1 -> Gain2/1
  Product/1 -> Gain/1
  Gain/1 -> F_t [N]/1
  Gain2/1 -> M_rot [Nm]/1
  Gain1/1 -> C_T/1

== system libturbines/Floating NREL5MW faulty/Aerodynamics/Blade 2 ==
  note: tip speed
      | [m/s]
  v_rot [m/s] : Inport
  beta [deg] : Inport  Port=2
  w_rot [rad/s] : Inport  Port=3
  C_P & C_T tables : Subsystem
  Gain : Gain  Gain=1/3
  Gain1 : Gain  Gain=1/3
  Gain2 : Gain  Gain=1/3
  Math Function : Math  Operator=square  SignedPower=on
  Product : Product  InputSameDT=on  SaturateOnIntegerOverflow=on  OutDataTypeStr=Inherit: Same as first input
  Product1 : Product  Inputs=**/  InputSameDT=on  SaturateOnIntegerOverflow=on  OutDataTypeStr=Inherit: Same as first input
  Product2 : Product  InputSameDT=on  SaturateOnIntegerOverflow=on  OutDataTypeStr=Inherit: Same as first input
  Product3 : Product  Inputs=/*  InputSameDT=on  SaturateOnIntegerOverflow=on  OutDataTypeStr=Inherit: Same as first input
  rho/2*A : Gain  Gain=env.rho*.5* pi * wt.rotor.radius^2  SaturateOnIntegerOverflow=on  OutDataTypeStr=Inherit: Same as input  ParamDataTypeStr=Inherit: Same as input
  rotor radius : Gain  Gain=wt.rotor.radius  SaturateOnIntegerOverflow=on  OutDataTypeStr=Inherit: Same as input  ParamDataTypeStr=Inherit: Same as input
  F_t [N] : Outport
  C_T : Outport  Port=2
  M_rot [Nm] : Outport  Port=3
  wires:
  C_P & C_T tables/2(C_P) -> Product1/1
  C_P & C_T tables/1(C_T) -> Gain1/1, Product/2
  Product3/1 -> C_P & C_T tables/2(lambda)
  rho/2*A/1 -> Product/1, Product2/2
  Product2/1 -> Product1/2
  w_rot [rad/s]/1 -> Product1/3, rotor radius/1
  v_rot [m/s]/1 -> Product2/1, Product3/1, Math Function/1
  rotor radius/1 -> Product3/2
  Math Function/1 -> rho/2*A/1
  beta [deg]/1 -> C_P & C_T tables/1(beta)
  Product1/1 -> Gain2/1
  Product/1 -> Gain/1
  Gain/1 -> F_t [N]/1
  Gain2/1 -> M_rot [Nm]/1
  Gain1/1 -> C_T/1

== system libturbines/Floating NREL5MW faulty/Aerodynamics/Blade 3 ==
  note: tip speed
      | [m/s]
  v_rot [m/s] : Inport
  beta [deg] : Inport  Port=2
  w_rot [rad/s] : Inport  Port=3
  C_P & C_T tables : Subsystem
  Gain : Gain  Gain=1/3
  Gain1 : Gain  Gain=1/3
  Gain2 : Gain  Gain=1/3
  Math Function : Math  Operator=square  SignedPower=on
  Product : Product  InputSameDT=on  SaturateOnIntegerOverflow=on  OutDataTypeStr=Inherit: Same as first input
  Product1 : Product  Inputs=**/  InputSameDT=on  SaturateOnIntegerOverflow=on  OutDataTypeStr=Inherit: Same as first input
  Product2 : Product  InputSameDT=on  SaturateOnIntegerOverflow=on  OutDataTypeStr=Inherit: Same as first input
  Product3 : Product  Inputs=/*  InputSameDT=on  SaturateOnIntegerOverflow=on  OutDataTypeStr=Inherit: Same as first input
  rho/2*A : Gain  Gain=env.rho*.5* pi * wt.rotor.radius^2  SaturateOnIntegerOverflow=on  OutDataTypeStr=Inherit: Same as input  ParamDataTypeStr=Inherit: Same as input
  rotor radius : Gain  Gain=wt.rotor.radius  SaturateOnIntegerOverflow=on  OutDataTypeStr=Inherit: Same as input  ParamDataTypeStr=Inherit: Same as input
  F_t [N] : Outport
  C_T : Outport  Port=2
  M_rot [Nm] : Outport  Port=3
  wires:
  C_P & C_T tables/2(C_P) -> Product1/1
  C_P & C_T tables/1(C_T) -> Gain1/1, Product/2
  Product3/1 -> C_P & C_T tables/2(lambda)
  rho/2*A/1 -> Product/1, Product2/2
  Product2/1 -> Product1/2
  w_rot [rad/s]/1 -> Product1/3, rotor radius/1
  v_rot [m/s]/1 -> Product2/1, Product3/1, Math Function/1
  rotor radius/1 -> Product3/2
  Math Function/1 -> rho/2*A/1
  beta [deg]/1 -> C_P & C_T tables/1(beta)
  Product1/1 -> Gain2/1
  Product/1 -> Gain/1
  Gain/1 -> F_t [N]/1
  Gain2/1 -> M_rot [Nm]/1
  Gain1/1 -> C_T/1

== system libturbines/Floating NREL5MW faulty/Controller/Pitch controller ==
  w_gen_diff : Inport
  P_dem : Inport  Port=2
  beta_meas [deg] : Inport  Port=3
  Enable : EnablePort  StatesWhenEnabling=reset  PropagateVarSize=During execution
  Blade 1 controller : Subsystem
  Blade 2 controller : Subsystem
  Blade 3 controller : Subsystem
  Demux : Demux  Outputs=3
  Mux : Mux  Inputs=3
  beta_ref [deg] : Outport  OutputWhenDisabled=reset  InitialOutput=wt.ctrl.torq.beta
  wires:
  Blade 2 controller/1(beta_ref [deg]) -> Mux/2
  Demux/3 -> Blade 3 controller/3(beta_meas [deg])
  Blade 3 controller/1(beta_ref [deg]) -> Mux/3
  beta_meas [deg]/1 -> Demux/1
  Demux/2 -> Blade 2 controller/3(beta_meas [deg])
  Blade 1 controller/1(beta_ref [deg]) -> Mux/1
  Demux/1 -> Blade 1 controller/3(beta_meas [deg])
  P_dem/1 -> Blade 3 controller/2(P_dem), Blade 2 controller/2(P_dem), Blade 1 controller/2(P_dem)
  w_gen_diff/1 -> Blade 3 controller/1(w_gen_diff), Blade 2 controller/1(w_gen_diff), Blade 1 controller/1(w_gen_diff)
  Mux/1 -> beta_ref [deg]/1
